simulink model "avlAerodynamics2D_th"  (R2018b)
settings: Solver=FixedStepAuto  StartTime=0.0  StopTime=0  RelTol=1e-3
values from neighbouring files (symbols this model uses):
  alpha = 0    [avlAerodynamics2D_ts2.m]
  beta = 0    [avlAerodynamics2D_ts2.m]
  defl = defls(ii)    [avlAerodynamics2D_ts2.m]
libraries: avlAerodynamics2D_ul x1
settings Model: Creator=mcobb  LastModifiedBy=mcobb

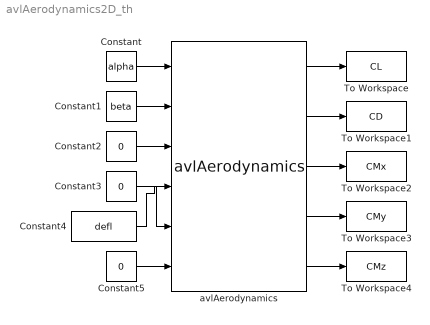
== system avlAerodynamics2D_th ==
  Constant : Constant  Value=alpha
  Constant1 : Constant  Value=beta
  Constant2 : Constant  Value=0
  Constant3 : Constant  Value=0
  Constant4 : Constant  Value=defl
  Constant5 : Constant  Value=0
  To Workspace : ToWorkspace  VariableName=CL  SaveFormat=Timeseries  SampleTime=-1
  To Workspace1 : ToWorkspace  VariableName=CD  SaveFormat=Timeseries  SampleTime=-1
  To Workspace2 : ToWorkspace  VariableName=CMx  SaveFormat=Timeseries  SampleTime=-1
  To Workspace3 : ToWorkspace  VariableName=CMy  SaveFormat=Timeseries  SampleTime=-1
  To Workspace4 : ToWorkspace  VariableName=CMz  SaveFormat=Timeseries  SampleTime=-1
  avlAerodynamics : avlAerodynamics2D_ul/avlAerodynamics  CLTable=CLtot_2D_Tbl  CDTable=CDtot_2D_Tbl  CMxTable=Cltot_2D_Tbl  CMyTable=Cmtot_2D_Tbl  CMzTable=Cntot_2D_Tbl  CS_gain=k_CS_gain
  wires:
  Constant1/1 -> avlAerodynamics/2
  Constant/1 -> avlAerodynamics/1
  Constant2/1 -> avlAerodynamics/3
  Constant3/1 -> avlAerodynamics/5
  Constant4/1 -> avlAerodynamics/4
  Constant5/1 -> avlAerodynamics/6
  avlAerodynamics/1 -> To Workspace/1
  avlAerodynamics/2 -> To Workspace1/1
  avlAerodynamics/3 -> To Workspace2/1
  avlAerodynamics/4 -> To Workspace3/1
  avlAerodynamics/5 -> To Workspace4/1
